simulink model "multikompar"  (R2012b)
settings: Solver=ode45  StartTime=0.0  StopTime=10.0  RelTol=1e-3
settings Model: Creator=Пользователь  LastModifiedBy=Jarda

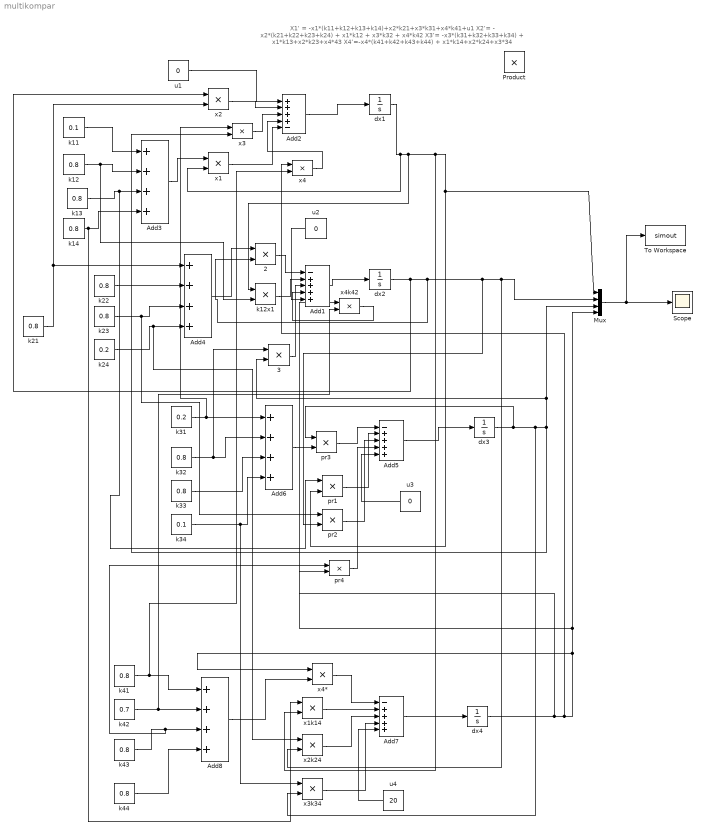
== system multikompar ==
  note: X1‘ = -x1*(k11+k12+k13+k14)+x2*k21+x3*k31+x4*k41+u1
      | X2’= - x2*(k21+k22+k23+k24) + x1*k12 + x3*k32 + x4*k42
      | X3’= -x3*(k31+k32+k33+k34) + x1*k13+x2*k23+x4*43
      | X4’=-x4*(k41+k42+k43+k44) + x1*k14+x2*k24+x3*34
  2 : Product  RndMeth=Zero
  3 : Product  RndMeth=Zero
  Add1 : Sum  Inputs=-++++
  Add2 : Sum  Inputs=++++-
  Add{3..4,6,8} (4 alike) : Sum  Inputs=++++
  Add5 : Sum  Inputs=-++++
  Add7 : Sum  Inputs=-++++
  Mux : Mux
  Product : Product  RndMeth=Zero
  Scope : Scope
  To Workspace : ToWorkspace  VariableName=simout  SampleTime=-1  SaveFormat=Timeseries
  dx1 : Integrator  InitialCondition=50
  dx2 : Integrator
  dx3 : Integrator
  dx4 : Integrator
  k11 : Constant  Value=0.1
  k{12..14,21..23,32..33,41,43..44} (11 alike) : Constant  Value=0.8
  k12x1 : Product  RndMeth=Zero
  k24 : Constant  Value=0.2
  k31 : Constant  Value=0.2
  k34 : Constant  Value=0.1
  k42 : Constant  Value=0.7
  pr{1..4} (4 alike) : Product  RndMeth=Zero
  u1 : Constant  Value=0
  u2 : Constant  Value=0
  u3 : Constant  Value=0
  u4 : Constant  Value=20
  x{1..4} (4 alike) : Product  RndMeth=Zero
  x1k14 : Product  RndMeth=Zero
  x2k24 : Product  RndMeth=Zero
  x3k34 : Product  RndMeth=Zero
  x4* : Product  RndMeth=Zero
  x4k42 : Product  RndMeth=Zero
  wires:
  Add2/1 -> dx1/1
  Mux/1 -> To Workspace/1, Scope/1
  dx2/1 -> x2/1, 2/2, pr2/2, x2k24/2, Mux/2
  u1/1 -> Add2/1
  x1/1 -> Add2/5
  Add3/1 -> x1/1
  k11/1 -> Add3/1
  k12/1 -> k12x1/2, Add3/2
  k13/1 -> pr1/1, Add3/3
  k14/1 -> x1k14/1, Add3/4
  x2/1 -> Add2/2
  k21/1 -> Add4/1, x2/2
  Add1/1 -> dx2/1
  Add4/1 -> 2/1
  k22/1 -> Add4/2
  k23/1 -> pr2/1, Add4/3
  k24/1 -> x2k24/1, Add4/4
  2/1 -> Add1/1
  k12x1/1 -> Add1/2
  3/1 -> Add1/3
  Add5/1 -> dx3/1
  k31/1 -> x3/1, Add6/1
  Add6/1 -> pr3/2
  pr3/1 -> Add5/1
  k32/1 -> 3/1, Add6/2
  k33/1 -> Add6/3
  k34/1 -> x3k34/1, Add6/4
  x3/1 -> Add2/3
  dx3/1 -> pr3/1, x3k34/2, Mux/3, 3/2, x3/2
  pr1/1 -> Add5/2
  dx1/1 -> x1/2, k12x1/1, x1k14/2, pr1/2, Mux/1
  pr2/1 -> Add5/3
  dx4/1 -> pr4/2, x4/1, x4k42/1, Mux/4, x4*/1
  Add7/1 -> dx4/1
  x4*/1 -> Add7/1
  Add8/1 -> x4*/2
  k44/1 -> Add8/4
  k43/1 -> pr4/1, Add8/3
  k42/1 -> x4k42/2, Add8/2
  k41/1 -> x4/2, Add8/1
  x1k14/1 -> Add7/2
  x2k24/1 -> Add7/3
  x3k34/1 -> Add7/4
  x4/1 -> Add2/4
  x4k42/1 -> Add1/4
  pr4/1 -> Add5/4
  u2/1 -> Add1/5
  u3/1 -> Add5/5
  u4/1 -> Add7/5
